simulink model "amp_mod"  (R2019b)
settings: Solver=VariableStepAuto  StartTime=0.0  StopTime=10.0  RelTol=1e-3
settings Model: Creator=LENOVO  LastModifiedBy=LENOVO

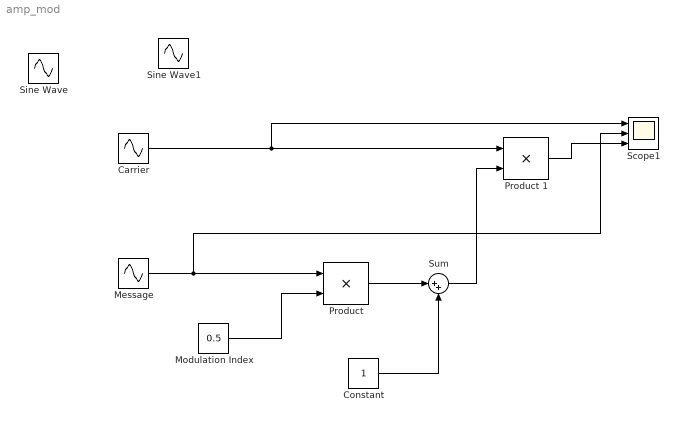
== system amp_mod ==
  Carrier : Sin  Frequency=2*pi*20  SampleTime=1/5000
  Constant : Constant
  Message : Sin  Frequency=2*pi*2  SampleTime=1/5000
  Modulation Index : Constant  Value=0.5
  "Product " : Product
  Product 1 : Product
  Scope1 : Scope  NumInputPorts=3
  Sine Wave : Sin  SampleTime=0
  Sine Wave1 : Sin  SampleTime=0
  Sum : Sum  Inputs=|++
  wires:
  Message/1 -> Scope1/2, "Product "/1
  Modulation Index/1 -> "Product "/2
  "Product "/1 -> Sum/1
  Constant/1 -> Sum/2
  Sum/1 -> Product 1/2
  Carrier/1 -> Scope1/1, Product 1/1
  Product 1/1 -> Scope1/3
